simulink model "Flanging"  (R2020b)
settings: Solver=VariableStepAuto  StartTime=0.0  StopTime=10.0  RelTol=1e-3
libraries: dspvision x1, dspsnks4 x1
settings Model: Creator=JonathanPC  LastModifiedBy=JonathanPC

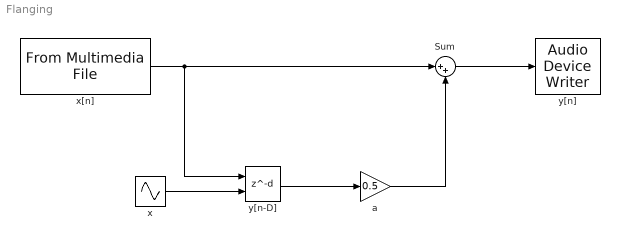
== system Flanging ==
  Sum : Sum  Inputs=|++
  a : Gain  Gain=0.5
  x : Sin  Amplitude=10  Frequency=25  SampleTime=0
  x[n] : dspvision/From Multimedia File  inputFilename=C:\Users\JonathanPC\Documents\MATLAB\taller2\Sonido.wav  readRange=[1 Inf]  loop=on  numPlays=inf  outputStreams=Audio only  videoDataType=single  audioDataType=double  inheritSampleTime=on  userDefinedSampleTime=1/30  noAudioOutput=off  isIntensityVideo=off  fourcc=RGB  colorVideoFormat=Separate color signals  outputEOF=off  dataOrg=Column-major  audioFrameSize=1024  computeAudioFrameSize=off  outSamplingMode=Sample based
  y[n-D] : Delay  DelayLengthSource=Input port
      settings: InputPortMap=u0,p1
  y[n] : dspsnks4/Audio Device Writer  Driver=DirectSound  Device=Default  InheritSampleRate=on  SampleRate=44100  BitDepth=16-bit integer  BufferSize=4096  NumBuffers=10  DefaultOutputChannelMapping=on  OutputChannelMapping=1:2  OutputNumUnderrunSamples=off  DriverIdx=1  DeviceWarnFlag=''
  wires:
  x[n]/1 -> y[n-D]/1, Sum/1
  Sum/1 -> y[n]/1
  a/1 -> Sum/2
  y[n-D]/1 -> a/1
  x/1 -> y[n-D]/2
